simulink model "sfun_build_02"  (R2013b)
settings: Solver=FixedStepDiscrete  StartTime=0.0  StopTime=30  FixedStep=0.01  RelTol=1e-3
settings Model: Creator=Administrator  LastModifiedBy=Administrator

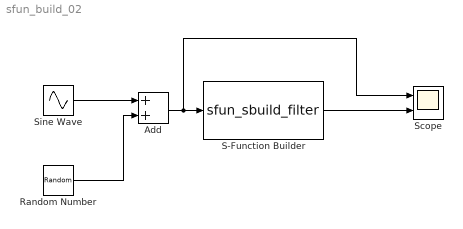
== system sfun_build_02 ==
  Add : Sum
  Random Number : RandomNumber
  S-Function Builder : S-Function  InitFcn=try, set_param(gcb,'FunctionName','sfun_sbuild_filter'), end  FunctionName=sfun_sbuild_filter  Parameters=0.005  SFunctionModules=sfun_sbuild_filter_wrapper  EnableBusSupport=off  mask(S-Function Builder){}
      mask help: Simulink:masks:SFunctionBuilder_MD
      mask init:
      | val = [[.9  0.75 0.75 1 1 .9 .9 1]',[1 1 0.75 0.75 .9 .9 1 .9]'];try , sys = get_param(gcb,'SfunBuilderFcnName');if isempty(sys), sys = get_param(gcb,'FunctionName'); end,catch, sys = get_param(gcb,'FunctionName'); end
      settings: CopyFcn=set_param(gcbh,'LinkStatus','none')  PreSaveFcn=try, set_param(gcb,'FunctionName','sfun_sbuild_filter'), end  OpenFcn=sfunctionwizard(gcbh)
      mask Display: plot(val(:,1),val(:,2)),disp(sys), port_label('input',1,'u'), port_label('output',1,'y')
  Scope : Scope  NumInputPorts=2
      settings: YMin=-5~-5  YMax=5~5
  Sine Wave : Sin
  wires:
  Sine Wave/1 -> Add/1
  Random Number/1 -> Add/2
  Add/1 -> Scope/1, S-Function Builder/1
  S-Function Builder/1 -> Scope/2
